simulink model "cv_2_sim"  (R2025b)
settings: Solver=VariableStepAuto  StartTime=0.0  StopTime=500  RelTol=1e-3
values from neighbouring files (symbols this model uses):
  mu = 0.62    [cv_2.m]
  rho = 1000    [cv_2.m]
  S = 1    [cv_2.m]
  S0 = 0.01    [cv_2.m]
undefined symbols (not defined in the file or in its folder): M1
settings Model: Creator=yehor  LastModifiedBy=yehor

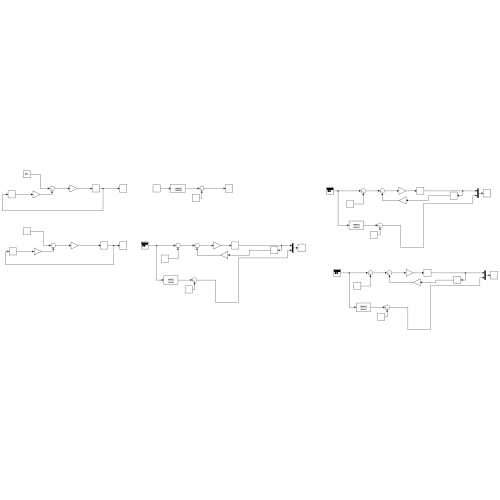
[thumbnail: Simulink's stored preview of the top-level diagram]
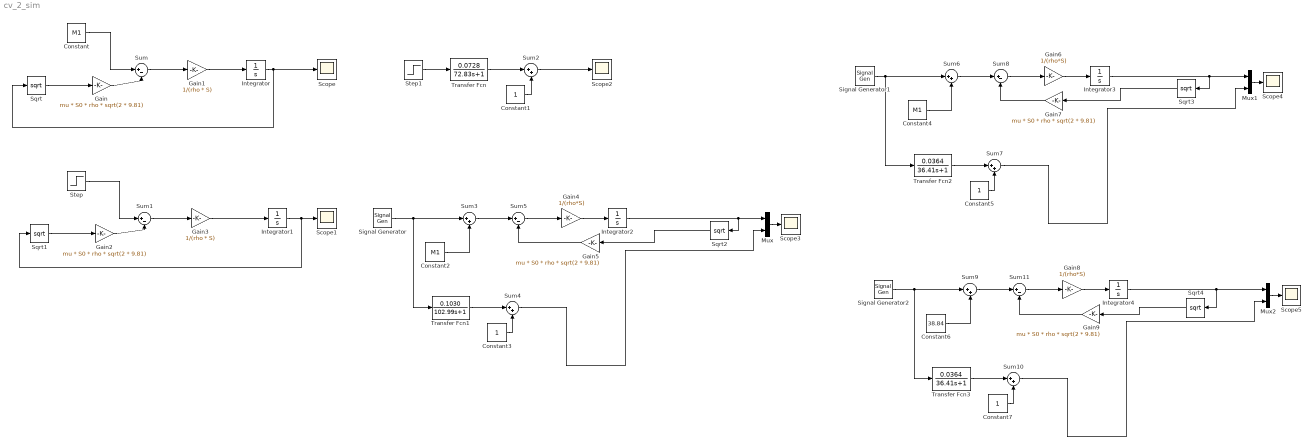
== system cv_2_sim ==
  Constant : Constant  Value=M1
  Constant{1,3,5,7} (4 alike) : Constant
  Constant2 : Constant  Value=M1
  Constant4 : Constant  Value=M1
  Constant6 : Constant  Value=38.84
  Gain{,2,5,7,9} (5 alike) : Gain  Gain=mu * S0 * rho * sqrt(2 * 9.81)
  Gain1 : Gain  Gain=1/(rho * S)
  Gain3 : Gain  Gain=1/(rho * S)
  Gain4 : Gain  Gain=1/(rho*S)
  Gain6 : Gain  Gain=1/(rho*S)
  Gain8 : Gain  Gain=1/(rho*S)
  Integrator{,2..4} (4 alike) : Integrator
  Integrator1 : Integrator  InitialCondition=1
  Mux : Mux  Inputs=2
  Mux1 : Mux  Inputs=2
  Mux2 : Mux  Inputs=2
  Scope{,1..5} (6 alike) : Scope
      Scope settings: ActiveDisplayYMinimum=-0.83521447085767475  ActiveDisplayYMaximum=1.4809268905417881
      Scope1 settings: ActiveDisplayYMinimum=-0.59451340619635074  ActiveDisplayYMaximum=1.2523332323758052
      Scope2 settings: ActiveDisplayYMinimum=-2.8765767768704551  ActiveDisplayYMaximum=1.6999481514865884  DataLoggingVariableName=ScopeData2
      Scope3 settings: ActiveDisplayYMinimum=-0.15506419983868225  ActiveDisplayYMaximum=1.3955777985481406  DataLoggingVariableName=ScopeData3
      Scope4 settings: ActiveDisplayYMinimum=-3.8234196581086821  ActiveDisplayYMaximum=34.410776922978144  DataLoggingVariableName=ScopeData4
      Scope5 settings: ActiveDisplayYMinimum=-4.91376354129957  ActiveDisplayYMaximum=44.22387187169614  DataLoggingVariableName=ScopeData5
  Signal Generator : SignalGenerator  WaveForm=square  Amplitude=5  Frequency=0.1571  Units=rad/sec
  Signal Generator1 : SignalGenerator  WaveForm=square  Amplitude=5  Frequency=0.1571  Units=rad/sec
  Signal Generator2 : SignalGenerator  WaveForm=square  Amplitude=5  Frequency=0.1571  Units=rad/sec
  Sqrt{,1..4} (5 alike) : Sqrt
  Step : Step  Time=0.01  Before=1  After=0  SampleTime=0
  Step1 : Step  Time=0.01  Before=1  After=-M1  SampleTime=0
  Sum{,1,5,8,11} (5 alike) : Sum  Inputs=|+-
  Sum{2..4,6..7,9..10} (7 alike) : Sum  Inputs=|++
  Transfer Fcn : TransferFcn  Numerator=[0.0728]  Denominator=[72.83 1]
  Transfer Fcn1 : TransferFcn  Numerator=[0.1030]  Denominator=[102.99 1]
  Transfer Fcn2 : TransferFcn  Numerator=[0.0364]  Denominator=[36.41 1]
  Transfer Fcn3 : TransferFcn  Numerator=[0.0364]  Denominator=[36.41 1]
  wires:
  Integrator/1 -> Sqrt/1, Scope/1
  Sqrt/1 -> Gain/1
  Gain/1 -> Sum/2
  Constant/1 -> Sum/1
  Sum/1 -> Gain1/1
  Step/1 -> Sum1/1
  Gain2/1 -> Sum1/2
  Integrator1/1 -> Scope1/1, Sqrt1/1
  Sqrt1/1 -> Gain2/1
  Sum1/1 -> Gain3/1
  Gain1/1 -> Integrator/1
  Gain3/1 -> Integrator1/1
  Step1/1 -> Transfer Fcn/1
  Transfer Fcn/1 -> Sum2/1
  Sum2/1 -> Scope2/1
  Constant1/1 -> Sum2/2
  Signal Generator/1 -> Transfer Fcn1/1, Sum3/1
  Constant2/1 -> Sum3/2
  Transfer Fcn1/1 -> Sum4/1
  Sum4/1 -> Mux/2
  Constant3/1 -> Sum4/2
  Sum3/1 -> Sum5/1
  Mux/1 -> Scope3/1
  Sum5/1 -> Gain4/1
  Gain4/1 -> Integrator2/1
  Sqrt2/1 -> Gain5/1
  Integrator2/1 -> Sqrt2/1, Mux/1
  Sum7/1 -> Mux1/2
  Sum8/1 -> Gain6/1
  Sqrt3/1 -> Gain7/1
  Signal Generator1/1 -> Transfer Fcn2/1, Sum6/1
  Sum6/1 -> Sum8/1
  Mux1/1 -> Scope4/1
  Gain6/1 -> Integrator3/1
  Constant4/1 -> Sum6/2
  Transfer Fcn2/1 -> Sum7/1
  Constant5/1 -> Sum7/2
  Sum11/1 -> Gain8/1
  Gain9/1 -> Sum11/2
  Signal Generator2/1 -> Transfer Fcn3/1, Sum9/1
  Transfer Fcn3/1 -> Sum10/1
  Sqrt4/1 -> Gain9/1
  Sum9/1 -> Sum11/1
  Sum10/1 -> Mux2/2
  Gain8/1 -> Integrator4/1
  Mux2/1 -> Scope5/1
  Constant6/1 -> Sum9/2
  Constant7/1 -> Sum10/2
  Gain5/1 -> Sum5/2
  Gain7/1 -> Sum8/2
  Integrator3/1 -> Sqrt3/1, Mux1/1
  Integrator4/1 -> Sqrt4/1, Mux2/1
